simulink model "test_model"  (R2020b)
settings: Solver=ode4  StartTime=0.0  StopTime=100  FixedStep=time_step  RelTol=1e-3
values from neighbouring files (symbols this model uses):
  A = [-0.05 1 0 ... (first row only)    [test.m]
  B = [2 ... (first row only)    [test.m]
  C = [0.5 0.5 0 ... (first row only)    [test.m]
  inputsize = inputsize(2)    [test.m]
  n = length(A)    [test.m]
  outputsize = outputsize(1)    [test.m]
  time_samples = 0:time_step:test_T    [test.m]
  time_samples_count = length(time_samples)    [test.m]
  time_step = 0.01    [test.m]
  x0 = ones(1, n)    [test.m]
undefined symbols (not defined in the file or in its folder): G1, G2, input_noise_power, output_noise_power
libraries: simulink x4
settings Model: Creator=Ja  LastModifiedBy=Mario
settings DebuggingCC: UnconnectedInputMsg=none  UnconnectedOutputMsg=none  UnconnectedLineMsg=none  SFMachineParentedDataDiag=error
settings ModelReferenceCC: EnableRefExpFcnMdlSchedulingChecks=off

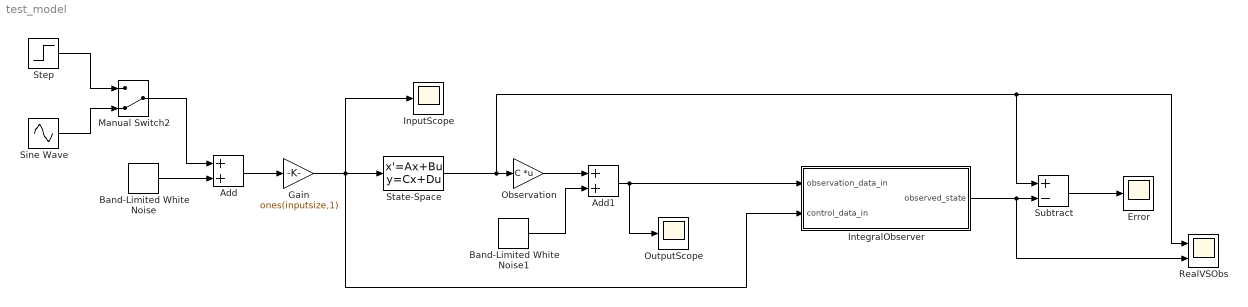
== system test_model ==
  Add : Sum
  Add1 : Sum
  Band-Limited White Noise : simulink/Sources/Band-Limited White Noise  Cov=[input_noise_power]  Ts=time_step  seed=[23341]
  Band-Limited White Noise1 : simulink/Sources/Band-Limited White Noise  Cov=[output_noise_power]  Ts=time_step  seed=[23341]
  Error : Scope
  Gain : Gain  Gain=ones(inputsize,1)
  InputScope : Scope
  IntegralObserver : Subsystem
  Manual Switch2 : ManualSwitch  CurrentSetting=0
  Observation : Gain  Gain=C  Multiplication=Matrix(K*u)
  OutputScope : Scope
  RealVSObs : Scope  NumInputPorts=2
  Sine Wave : Sin  SampleTime=0
  State-Space : StateSpace  A=A  B=B  C=eye(n)  D=zeros(n, inputsize)  InitialCondition=x0
  Step : Step  Time=3  SampleTime=0
  Subtract : Sum  Inputs=+-
  wires:
  Add1/1 -> OutputScope/1, IntegralObserver/1(observation_data_in)
  State-Space/1 -> RealVSObs/1, Subtract/1, Observation/1
  Band-Limited White Noise/1 -> Add/2
  Band-Limited White Noise1/1 -> Add1/2
  Observation/1 -> Add1/1
  Step/1 -> Manual Switch2/1
  Sine Wave/1 -> Manual Switch2/2
  Manual Switch2/1 -> Add/1
  Subtract/1 -> Error/1
  Gain/1 -> IntegralObserver/2(control_data_in), InputScope/1, State-Space/1
  Add/1 -> Gain/1
  IntegralObserver/1(observed_state) -> Subtract/2, RealVSObs/2

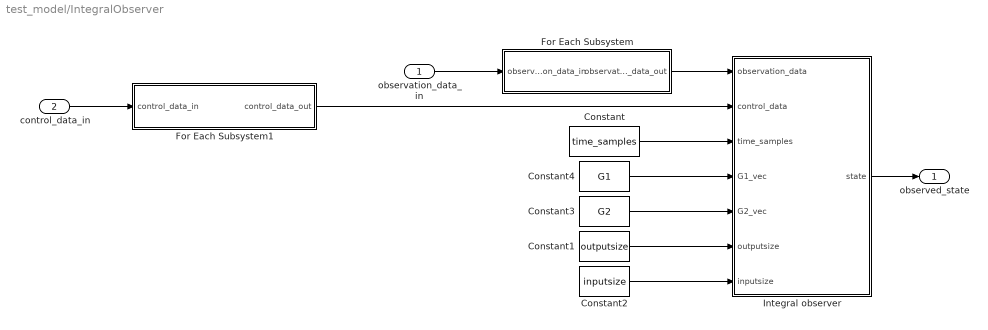
== system test_model/IntegralObserver ==
  observation_data_in : Inport
  control_data_in : Inport  Port=2
  Constant : Constant  Value=time_samples
  Constant1 : Constant  Value=outputsize
  Constant2 : Constant  Value=inputsize
  Constant3 : Constant  Value=G2
  Constant4 : Constant  Value=G1
  For Each Subsystem : Subsystem  TreatAsAtomicUnit=on
  For Each Subsystem1 : Subsystem  TreatAsAtomicUnit=on
  Integral observer : MATLAB Function  TreatAsAtomicUnit=on
  observed_state : Outport
  wires:
  Constant3/1 -> Integral observer/5(G2_vec)
  For Each Subsystem/1(observation_data_out) -> Integral observer/1(observation_data)
  Constant2/1 -> Integral observer/7(inputsize)
  Constant4/1 -> Integral observer/4(G1_vec)
  control_data_in/1 -> For Each Subsystem1/1(control_data_in)
  Constant1/1 -> Integral observer/6(outputsize)
  For Each Subsystem1/1(control_data_out) -> Integral observer/2(control_data)
  Constant/1 -> Integral observer/3(time_samples)
  Integral observer/1(state) -> observed_state/1
  observation_data_in/1 -> For Each Subsystem/1(observation_data_in)

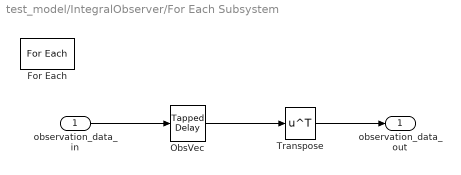
== system test_model/IntegralObserver/For Each Subsystem ==
  observation_data_in : Inport  Partition=on  PartitionDimension=1  PartitionWidth=1  PartitionOffset=0
  For Each : ForEach  DisableCoverage=on
  ObsVec : simulink/Discrete/Tapped Delay  vinit=0.0  samptime=-1  NumDelays=time_samples_count  DelayOrder=Oldest  includeCurrent=off
  Transpose : Math  Operator=transpose  SaturateOnIntegerOverflow=on
  observation_data_out : Outport  ConcatenationDimension=1
  wires:
  observation_data_in/1 -> ObsVec/1
  ObsVec/1 -> Transpose/1
  Transpose/1 -> observation_data_out/1

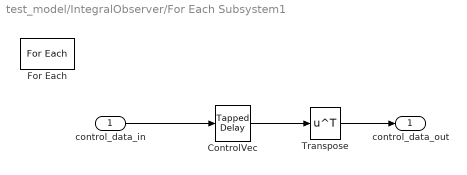
== system test_model/IntegralObserver/For Each Subsystem1 ==
  control_data_in : Inport  Partition=on  PartitionDimension=1  PartitionWidth=1  PartitionOffset=0
  ControlVec : simulink/Discrete/Tapped Delay  vinit=0.0  samptime=-1  NumDelays=time_samples_count  DelayOrder=Oldest  includeCurrent=off
  For Each : ForEach  DisableCoverage=on
  Transpose : Math  Operator=transpose  SaturateOnIntegerOverflow=on
  control_data_out : Outport  ConcatenationDimension=1
  wires:
  control_data_in/1 -> ControlVec/1
  ControlVec/1 -> Transpose/1
  Transpose/1 -> control_data_out/1

== matlab function test_model/IntegralObserver/Integral observer ==
  data: observation_data input; state output size=n; control_data input; time_samples input; G1_vec input; G2_vec input; outputsize input; inputsize input
function state = fcn(observation_data, control_data, time_samples,G1_vec, G2_vec, outputsize, inputsize)
    % funkcja licząca numerycznie obserwacje
    
    G1xY = squeeze(sum(bsxfun(@mtimes,G1_vec,reshape(observation_data, 1, outputsize, [])),2));
    G2xU = squeeze(sum(bsxfun(@mtimes,G2_vec,reshape(control_data, 1, inputsize, [])),2));
    
    state_obs = trapz(time_samples, G1xY, 2);
    control_obs = trapz(time_samples, G2xU, 2);
    
    state = state_obs + control_obs;
end
